simulink model "lab2"  (R2015b)
settings: Solver=FixedStepDiscrete  StartTime=0.0  StopTime=100.0  RelTol=1e-3
undefined symbols (not defined in the file): DiscIntNeverNeededParam
settings Model: Creator=Администратор  LastModifiedBy=Администратор

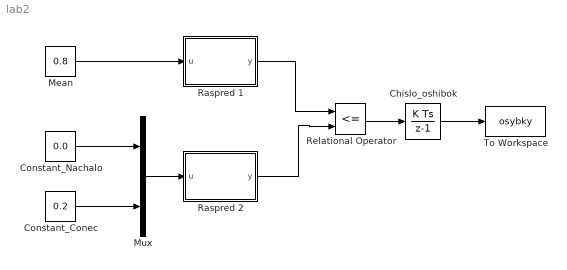
== system lab2 ==
  Chislo_oshibok : DiscreteIntegrator  InitialConditionSetting=State (most efficient)  ICPrevOutput=DiscIntNeverNeededParam  ICPrevScaledInput=DiscIntNeverNeededParam
  Constant_Conec : Constant  Value=0.2
  Constant_Nachalo : Constant  Value=0.0
  Mean : Constant  Value=0.8
  Mux : Mux  Inputs=2
  Raspred 1 : MATLAB Function  TreatAsAtomicUnit=on
  Raspred 2 : MATLAB Function  TreatAsAtomicUnit=on
  Relational Operator : RelationalOperator  Operator=<=  OutDataTypeStr=boolean
  To Workspace : ToWorkspace  VariableName=osybky  SaveFormat=Timeseries  SampleTime=-1
  wires:
  Mean/1 -> Raspred 1/1(u)
  Constant_Nachalo/1 -> Mux/1
  Constant_Conec/1 -> Mux/2
  Mux/1 -> Raspred 2/1(u)
  Raspred 1/1(y) -> Relational Operator/1
  Raspred 2/1(y) -> Relational Operator/2
  Relational Operator/1 -> Chislo_oshibok/1
  Chislo_oshibok/1 -> To Workspace/1

== matlab function lab2/Raspred 2 ==
  data: u input; y output
function y = fcn(u)
coder.extrinsic('unifrnd','rng');
y = 0;
persistent atTime0
if isempty(atTime0)
rng('shuffle');
atTime0 = false;
end
y = unifrnd(u(1),u(2),1,1);

== matlab function lab2/Raspred 1 ==
  data: u input; y output
function y = fcn(u)
coder.extrinsic('exprnd','rng');
y = 0;
persistent atTime0
if isempty(atTime0)
rng('shuffle');
atTime0 = false;
end
y = exprnd(u,1,1);
